simulink model "lab3_05_gain_compare_slx"  (R2025b)
settings: Solver=ode45  StartTime=0.0  StopTime=10.0  MaxStep=0.01  RelTol=1e-6
settings Model: Creator=Boris  LastModifiedBy=Boris

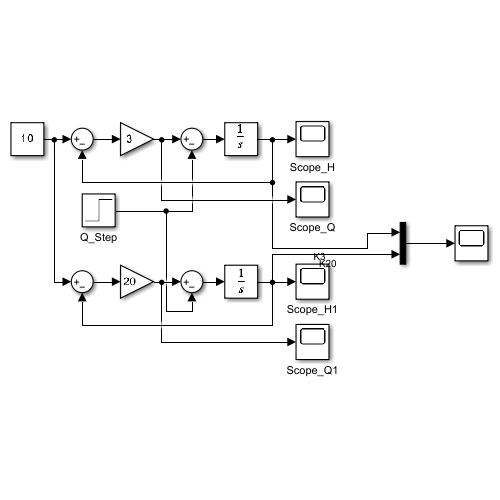
[thumbnail: Simulink's stored preview of the top-level diagram]
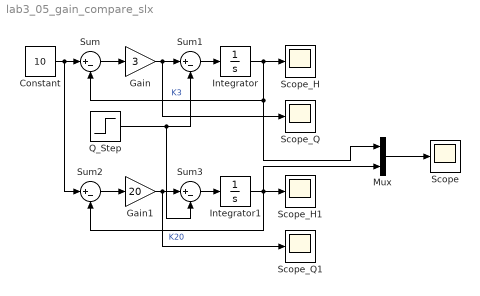
== system lab3_05_gain_compare_slx ==
  Constant : Constant  Value=10
  Gain : Gain  Gain=3
  Gain1 : Gain  Gain=20
  Integrator : Integrator
  Integrator1 : Integrator
  Mux : Mux  Inputs=2
  Q_Step : Step  Time=6  After=2  SampleTime=0
  Scope : Scope
      settings: ActiveDisplayYMinimum=6.0085097848368179  ActiveDisplayYMaximum=11.059154766282987  DataLoggingVariableName=ScopeData4
  Scope_H : Scope
      settings: ActiveDisplayYMinimum=-12.737485297214677  ActiveDisplayYMaximum=18.6045938448039
  Scope_H1 : Scope
      settings: ActiveDisplayYMinimum=-12.737485297214677  ActiveDisplayYMaximum=18.6045938448039  DataLoggingVariableName=ScopeData2
  Scope_Q : Scope
      settings: ActiveDisplayYMinimum=-13.964369062402058  ActiveDisplayYMaximum=20.590273191673429
  Scope_Q1 : Scope
      settings: ActiveDisplayYMinimum=-13.964369062402058  ActiveDisplayYMaximum=20.590273191673429  DataLoggingVariableName=ScopeData3
  Sum{,1..3} (4 alike) : Sum  Inputs=|+-
  wires:
  Integrator/1 -> Mux/1, Sum/2, Scope_H/1  "K3"
  Sum/1 -> Gain/1
  Gain/1 -> Scope_Q/1, Sum1/1
  Sum1/1 -> Integrator/1
  Q_Step/1 -> Sum1/2, Sum3/2
  Gain1/1 -> Scope_Q1/1, Sum3/1
  Constant/1 -> Sum2/1, Sum/1
  Sum3/1 -> Integrator1/1
  Integrator1/1 -> Mux/2, Sum2/2, Scope_H1/1  "K20"
  Sum2/1 -> Gain1/1
  Mux/1 -> Scope/1
